simulink model "linearmodel"  (R2020a)
settings: Solver=FixedStepAuto  StartTime=0.0  StopTime=1.3  FixedStep=0.001  RelTol=1e-3
undefined symbols (not defined in the file or in its folder): c, k, m
libraries: simulink x1
settings Model: Creator=User  LastModifiedBy=User

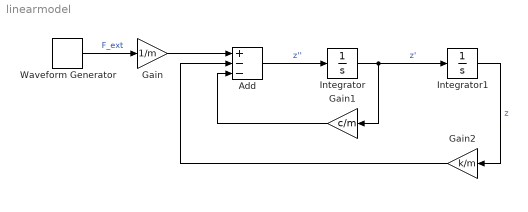
== system linearmodel ==
  Add : Sum  Inputs=+--
  Gain : Gain  Gain=1/m
  Gain1 : Gain  Gain=c/m
  Gain2 : Gain  Gain=k/m
  Integrator : Integrator
  Integrator1 : Integrator
  Waveform Generator : simulink/Sources/Waveform Generator  OutMin=[]  OutMax=[]  OutDataTypeStr=double  SelectedSignal=1  BlockNames=MultiportSwitch_e3df3653d217406  SampleTime=0.1
  wires:
  Integrator/1 -> Gain1/1, Integrator1/1  "z'"
  Integrator1/1 -> Gain2/1  "z"
  Add/1 -> Integrator/1  "z''"
  Gain1/1 -> Add/3
  Gain/1 -> Add/1
  Waveform Generator/1 -> Gain/1  "F_ext"
  Gain2/1 -> Add/2
